simulink library "MX_Library"  (Simulink 7.7)
settings: Solver=ode45  StartTime=0.0  StopTime=10.0  RelTol=1e-3
values from neighbouring files (symbols this model uses):
  ACTIVE = Bobcat.Parameter; CreateDefine( ACTIVE                         ,1                          ,'Define' ,'defines.h' )    [defines.m]
  CD_PRECISION_REF_NOMINAL_VALUE = Bobcat.Parameter; CreateAliasCD( CD_PRECISION_REF_NOMINAL_VALUE                       ,uint16(511)                ,'ConstantDataPointer' ,'CONSTANT_DATA' ,'PRECISION_REF_NOMINAL_VALUE')    [cdata.m]
  ENGINE_CRANKING = Bobcat.Parameter; CreateDefine( ENGINE_CRANKING                ,2                          ,'Define' ,'defines.h' )    [defines.m]
  ERROR_OFF = Bobcat.Parameter; CreateDefine( ERROR_OFF                      ,3                          ,'Define' ,'defines.h' )    [defines.m]
  ERROR_ON = Bobcat.Parameter; CreateDefine( ERROR_ON                       ,2                          ,'Define' ,'defines.h' )    [defines.m]
  FAILURE = Bobcat.Parameter; CreateDefine( FAILURE                        ,28                         ,'Define' ,'defines.h' )    [defines.m]
  FULL_ON = Bobcat.Parameter; CreateDefine( FULL_ON                        ,fi(0,0,16,16,'hex','ffff') ,'Define' ,'defines.h' )    [defines.m]
  INACTIVE = Bobcat.Parameter; CreateDefine( INACTIVE                       ,0                          ,'Define' ,'defines.h' )    [defines.m]
  NON_FUNCTIONAL = Bobcat.Parameter; CreateDefine( NON_FUNCTIONAL                 ,255                        ,'Define' ,'defines.h' )    [defines.m]
  NORMAL = Bobcat.Parameter; CreateDefine( NORMAL                         ,8                          ,'Define' ,'defines.h' )    [defines.m]
  OORL = Bobcat.Parameter; CreateDefine( OORL                           ,22                         ,'Define' ,'defines.h' )    [defines.m]
  OPEN_CIRCUIT = Bobcat.Parameter; CreateDefine( OPEN_CIRCUIT                   ,7                          ,'Define' ,'defines.h' )    [defines.m]
  OPEN_STG = Bobcat.Parameter; CreateDefine( OPEN_STG                       ,31                         ,'Define' ,'defines.h' )    [defines.m]
  OVERCURRENT = Bobcat.Parameter; CreateDefine( OVERCURRENT                    ,32                         ,'Define' ,'defines.h' )    [defines.m]
  RESET = Bobcat.Parameter; CreateDefine( RESET                          ,2                          ,'Define' ,'defines.h' )    [defines.m]
  SHORT_TO_BATTERY = Bobcat.Parameter; CreateDefine( SHORT_TO_BATTERY               ,5                          ,'Define' ,'defines.h' )    [defines.m]
  SHORT_TO_GROUND = Bobcat.Parameter; CreateDefine( SHORT_TO_GROUND                ,6                          ,'Define' ,'defines.h' )    [defines.m]
  srate = 0.010    (= 0.01)    [LoadWorkspace.m]
  UNLIMITED = Bobcat.Parameter; CreateDefine( UNLIMITED                      ,65535                      ,'Define' ,'defines.h' )    [defines.m]
undefined symbols (not defined in the file or in its folder): BIDIRECTIONAL_CTRL, CD__AFBK_GAIN, CD__DEBOUNCE_OPEN_CIRCUIT, CD__DEBOUNCE_OVERCURRENT, CD__DEBOUNCE_SHORT_TO_BATTERY, CD__DEBOUNCE_SHORT_TO_GROUND, CD__ENABLE_AFBK_GAIN, CD__ENABLE_DEBOUNCE_OPEN_CIRCUIT, CD__ENABLE_DEBOUNCE_OVERCURRENT, CD__ENABLE_DEBOUNCE_SHORT_TO_BATTERY, CD__ENABLE_DEBOUNCE_SHORT_TO_GROUND, CD__ENABLE_FEEDBACK_FUNCTION, CD__ENABLE_IFBK_GAIN, CD__ENABLE_MAX_VOLTS, CD__ENABLE_NON_ZERO_CURRENT, CD__ENABLE_NON_ZERO_DUTY, CD__ENABLE_OVERCURRENT, CD__FUNCTION, CD__IFBK_GAIN, CD__KI, CD__KP, CD__MAX_VOLTS, CD__NON_ZERO_CURRENT, CD__NON_ZERO_DUTY, CD__OVERCURRENT, DEBOUNCE_ERROR_OFF, DEBOUNCE_ERROR_ON, DiscIntNeverNeededParam, FN_, IFBK_MAX, KI, KP, MAX_VOLTS, NZ_DUTY, NZ_IFBK, OC_DB_CNT, OPEN_DB_CNT, OSTG_DB_CNT, STB_DB_CNT, STG_DB_CNT
libraries: simulink x12, MX_Library x11
(part 2 of 2)

== stateflow chart oc_stg_detection/oc_operation_detection ==
  state NORMAL
    en:diag_state_out = NORMAL;
    en:ocstg_check = INACTIVE;
  state OC_STATE_ERROR
    en:diag_state_out = oc_state;
    en:ocstg_check = INACTIVE;
  state OPEN_STG_ERROR_RESET
    en:diag_state_out = NORMAL;
    en:ocstg_check = ACTIVE;
  state OPEN_STG_ERROR
    du:diag_state_out = diag_state_in;
    en:ocstg_check = INACTIVE;
    en:debounceCount = 0;
    (junction 157) -> (junction 158) : [(diag_state_in == NORMAL)]{debounceCount++;}
    OPEN_STG_ERROR -> (junction 157) [order 1]
  state DIAG_STATE_ERROR
    en:diag_state_out = diag_state_in;
    en:ocstg_check = INACTIVE;
  state OPEN_STG_DIAG_STATE
    en:ocstg_check = INACTIVE;
  state OPEN_STG_RESET
    en:ocstg_check = RESET;
  note: Pulse ocstg_check to reset fault state
      | to normal with output forced off to determine
      | if the fault is STG or Open Circuit
  note: During this state, lo-side is to enabled for a period of time to determine
      | if fault is open circuit.  Then lo-side is to be turned off to check for
      | short to ground.
  note: Error no longer detectable,
      | send reset to turn the output back on.
  (default) -> NORMAL
  NORMAL -> OPEN_STG_ERROR_RESET [order 1] : %Unable to distinguish
      | % between Open or STG fault
      | [(diag_state_in == OPEN_STG)]
  NORMAL -> OC_STATE_ERROR [order 2] : %Overcurrent Fault
      | [(oc_state != NORMAL)]
  OPEN_STG_DIAG_STATE -> OPEN_STG_ERROR : [after(5,tick)]
  NORMAL -> DIAG_STATE_ERROR [order 3] : %STB, STG or Open Circuit Fault
      | [(diag_state_in == SHORT_TO_GROUND)...
      | || (diag_state_in == SHORT_TO_BATTERY)...
      | || (diag_state_in == OPEN_CIRCUIT)]
  OPEN_STG_ERROR_RESET -> OPEN_STG_DIAG_STATE : [after(5,tick)]
  OPEN_STG_RESET -> NORMAL : [after(50,tick)]
  OPEN_STG_ERROR -> OPEN_STG_RESET [order 1] : [(debounceCount >= (OPEN_DB_CNT...
      | + STG_DB_CNT + 100))]
  data: oc_state input uint8; diag_state_in input uint8; diag_state_out output uint8; ocstg_check output uint8; ACTIVE parameter uint8; INACTIVE parameter uint8; OPEN_CIRCUIT parameter uint8; SHORT_TO_GROUND parameter uint8; SHORT_TO_BATTERY parameter uint8; OPEN_STG parameter uint8; NORMAL parameter uint8; debounceCount local uint16; RESET parameter uint8; OPEN_DB_CNT parameter uint16; STG_DB_CNT parameter uint16

== stateflow chart output_pair_ClosedLoop/control ==
  state DIAG_CHECK
    en:icmd_Out = INACTIVE;
    state ENABLE_ON
      en:enable_LoSide = ACTIVE;
      en:debounceCount = 0;
      du:debounceCount++;
    state ENABLE_OFF
      en:enable_LoSide = INACTIVE;
    note: Turns on the low side
        | (may take up to 0.5 sec for low side to actually
        | turn on due to delay in output enable function).
        | So, it is possible to detect STG right away
        | while in this state.
    note: Forces the low side off for STG detection
        | assuming it didn't detect it already while
        | waiting for the low side to turn on.
    note: To detect open circuit, low side must be on.
        | To detect STG, low side must be off.
    (default) -> ENABLE_ON
    ENABLE_ON -> ENABLE_OFF : %Give it some time to ensure low side is on
        | %and detect open circuit
        | [(debounceCount >= OPEN_DB_CNT + 100)]
  state ERROR
    en:
    icmd_Out = INACTIVE;
    enable_LoSide = INACTIVE;
    state_Output = diag_state;
  state FUNCTIONAL
    state STGOFF_DIAG_ACTIVE
      en:icmd_Out = INACTIVE;
      en:state_Output = INACTIVE;
      state Test_OC
        en:debounceCount = 0;
        en:enable_LoSide = ACTIVE;
        du:debounceCount++;
      state Test_STG
        en:debounceCount = 0;
        en:enable_LoSide = INACTIVE;
        du:debounceCount++;
      note: Testing for open circuit will turn on the low side
          | (may take up to 0.5 sec for low side to actually
          | turn on due to delay in output enable function).
          | So, it is possible to detect STG right away
          | while in this state.
      note: Forces the low side off for STG detection
          | assuming it didn't detect it already while
          | waiting for the low side to turn on.
      (default) -> Test_OC
      Test_STG -> Test_OC : [(debounceCount >= STG_DB_CNT + 100)]
      Test_OC -> Test_STG : [(debounceCount >= OPEN_DB_CNT + 100)]
    state STGOFF_DIAG_INACTIVE
      en:enable_LoSide = ACTIVE;
      state ACTIVE_ON
        en:icmd_Out = icmd_In;
        du:icmd_Out = icmd_In;
        en:state_Output = ACTIVE;
      state ACTIVE_OFF
        en:icmd_Out = INACTIVE;
        en:state_Output = INACTIVE;
      (default) -> ACTIVE_OFF
      ACTIVE_ON -> ACTIVE_OFF : [icmd_In == 0]
      ACTIVE_OFF -> ACTIVE_ON : [icmd_In > 0]
    note: Short to Ground detection is available
        | while hi side output is off by turning
        | off low-side periodically.
    note: Short to Ground detection is
        | not available while hi side output
        | is off
    STGOFF_DIAG_ACTIVE -> STGOFF_DIAG_INACTIVE : [!enable_STGOffDiag]
    STGOFF_DIAG_INACTIVE -> STGOFF_DIAG_ACTIVE : [enable_STGOffDiag]
    (default) -> STGOFF_DIAG_ACTIVE
  DIAG_CHECK -> FUNCTIONAL [order 1] : %Couldn't find a fault, so go back to working
      | %?? should this condition really be recoverable??
      | [(ocstg_check == RESET)]
  FUNCTIONAL -> DIAG_CHECK [order 2] : %Open or STG Fault detected
      | %while output is on
      | [(ocstg_check == ACTIVE)]
  (default) -> FUNCTIONAL
  DIAG_CHECK -> ERROR [order 2] : %Fault Detected
      | [(diag_state != NORMAL)]
  FUNCTIONAL -> ERROR [order 1] : %Fault Detected
      | [(diag_state != NORMAL)]
  data: state_Output output uint8; icmd_In input fixdt(0,16,12); icmd_Out output fixdt(0,16,12); enable_LoSide output boolean; ocstg_check input uint8; debounceCount local uint16 =0; ACTIVE parameter uint8; INACTIVE parameter uint8; RESET parameter uint8; diag_state input uint8; NORMAL parameter uint8; OPEN_DB_CNT parameter uint16; STG_DB_CNT parameter uint16; enable_STGOffDiag input boolean

== stateflow chart output_single_OpenLoop/control ==
  state ERROR
    en:duty_Output = INACTIVE;
    en:state_Output = error_Output;
  state FUNCTIONAL
    en:
    duty_Output = cmd_Output;
    du:
    duty_Output = cmd_Output;
    state ACTIVE
      en:
      state_Output = ACTIVE;
    state INACTIVE
      en:
      state_Output = INACTIVE;
    INACTIVE -> ACTIVE : [cmd_Output != INACTIVE]
    (default) -> INACTIVE
    ACTIVE -> INACTIVE : [cmd_Output == INACTIVE]
  FUNCTIONAL -> ERROR : [(error_Output != NORMAL)]
  ERROR -> FUNCTIONAL : [(error_Output == NORMAL)]
  (default) -> FUNCTIONAL
  data: duty_Output output fixdt(0,16,16); state_Output output uint8; cmd_Output input fixdt(0,16,16); error_Output input uint8; INACTIVE parameter uint8 =0; ACTIVE parameter uint8 =1; NORMAL parameter uint8

== stateflow chart output_pair_OpenLoop/control ==
  state DIAG_CHECK
    en:duty_Output = INACTIVE;
    state ENABLE_ON
      en:enable_LoSide = ACTIVE;
      en:debounceCount = 0;
      du:debounceCount++;
    state ENABLE_OFF
      en:enable_LoSide = INACTIVE;
    note: Turns on the low side
        | (may take up to 0.5 sec for low side to actually
        | turn on due to delay in output enable function).
        | So, it is possible to detect STG right away
        | while in this state.
    note: Forces the low side off for STG detection
        | assuming it didn't detect it already while
        | waiting for the low side to turn on.
    note: To detect open circuit, low side must be on.
        | To detect STG, low side must be off.
    (default) -> ENABLE_ON
    ENABLE_ON -> ENABLE_OFF : %Give it some time to ensure low side is on
        | %and detect open circuit
        | [(debounceCount >= OPEN_DB_CNT + 100)]
  state ERROR
    en:
    duty_Output = INACTIVE;
    enable_LoSide = INACTIVE;
    state_Output = diag_state;
  state FUNCTIONAL
    state STGOFF_DIAG_ACTIVE
      en:duty_Output = INACTIVE;
      en:state_Output = INACTIVE;
      state Test_OC
        en:debounceCount = 0;
        en:enable_LoSide = ACTIVE;
        du:debounceCount++;
      state Test_STG
        en:debounceCount = 0;
        en:enable_LoSide = INACTIVE;
        du:debounceCount++;
      note: Testing for open circuit will turn on the low side
          | (may take up to 0.5 sec for low side to actually
          | turn on due to delay in output enable function).
          | So, it is possible to detect STG right away
          | while in this state.
      note: Forces the low side off for STG detection
          | assuming it didn't detect it already while
          | waiting for the low side to turn on.
      (default) -> Test_OC
      Test_STG -> Test_OC : [(debounceCount >= STG_DB_CNT + 100)]
      Test_OC -> Test_STG : [(debounceCount >= OPEN_DB_CNT + 100)]
    state STGOFF_DIAG_INACTIVE
      en:enable_LoSide = ACTIVE;
      state ACTIVE_ON
        en:duty_Output = FULL_ON;
        en:state_Output = ACTIVE;
      state ACTIVE_OFF
        en:duty_Output = INACTIVE;
        en:state_Output = INACTIVE;
      (default) -> ACTIVE_OFF
      ACTIVE_ON -> ACTIVE_OFF : [(cmd_Output != ACTIVE)]
      ACTIVE_OFF -> ACTIVE_ON : [(cmd_Output == ACTIVE)]
    note: Short to Ground detection is available
        | while hi side output is off by turning
        | off low-side periodically.
    note: Short to Ground detection is
        | not available while hi side output
        | is off
    STGOFF_DIAG_ACTIVE -> STGOFF_DIAG_INACTIVE : [!enable_STGOffDiag]
    STGOFF_DIAG_INACTIVE -> STGOFF_DIAG_ACTIVE : [enable_STGOffDiag]
    (default) -> STGOFF_DIAG_ACTIVE
  DIAG_CHECK -> FUNCTIONAL [order 1] : %Couldn't find a fault, so go back to working
      | %?? should this condition really be recoverable??
      | [(ocstg_check == RESET)]
  FUNCTIONAL -> DIAG_CHECK [order 2] : %Open or STG Fault detected
      | %while output is on
      | [(ocstg_check == ACTIVE)]
  (default) -> FUNCTIONAL
  DIAG_CHECK -> ERROR [order 2] : %Fault Detected
      | [(diag_state != NORMAL)]
  FUNCTIONAL -> ERROR [order 1] : %Fault Detected
      | [(diag_state != NORMAL)]
  ERROR -> FUNCTIONAL : [(diag_state == NORMAL)]
  data: state_Output output uint8; cmd_Output input boolean; enable_STGOffDiag input boolean; duty_Output output fixdt(0,16,16); enable_LoSide output boolean; ocstg_check input uint8; debounceCount local uint16 =0; ACTIVE parameter uint8; INACTIVE parameter uint8; RESET parameter uint8; diag_state input uint8; NORMAL parameter uint8; OPEN_DB_CNT parameter uint16; STG_DB_CNT parameter uint16; FULL_ON parameter fixdt(0,16,16)

== stateflow chart dout_chk/Fault monitor ==
  state diagnostics
    during: os=out_state();
    state Ok
      en: state = 8;
    state error
      en: state=os;
    state debounce
    state y=out_state [function]
      (default) -> (junction 314)
      (junction 314) -> (junction 315) : {
          | /* command, off feedback, on */
          | aVarTruthTableCondition_1 = (cmd==0 && fbk==1);
          | }
      (junction 315) -> (junction 316) : {
          | /* command, on feedback, off */
          | aVarTruthTableCondition_2 = (cmd==1 && fbk==0);
          | }
      (junction 316) -> (junction 317) [order 1] : [aVarTruthTableCondition_1]
      (junction 317) -> (junction 318) : {
          | /* 'E_on':Error On */
          | y=2; db_limit=ERR_ON_DB_CNT;
          | }
      (junction 316) -> (junction 319) [order 2]
      (junction 319) -> (junction 320) [order 1] : [aVarTruthTableCondition_2]
      (junction 320) -> (junction 321) : {
          | /* 'E_off':Error Off */
          | y=3; db_limit=ERR_OFF_DB_CNT;
          | }
      (junction 319) -> (junction 322) [order 2]
      (junction 322) -> (junction 323) : /* Default */
      (junction 323) -> (junction 324) : {
          | /* 'ok':default */
          | y=8;
          | }
    (default) -> Ok
    debounce -> error [order 2] : [db_cnt >= db_limit]
    debounce -> (junction 313) [order 3]
    debounce -> Ok [order 1] : [db_cnt==0]
    Ok -> debounce : [os!=8]/
        | db_state=os;
        | db_cnt++;
    (junction 312) -> debounce [order 2] : {db_cnt=1;
        | db_state=os}
    (junction 313) -> debounce [order 1] : [db_state==os]/
        | db_cnt++;
    (junction 313) -> (junction 312) [order 2]
    (junction 312) -> debounce [order 1] : [os==8]/
        | db_cnt--;
  data: os local uint8; db_cnt local uint16; db_state local uint8; db_limit local uint16 =20; y function_output uint8; aVarTruthTableCondition_1 temporary boolean =0; aVarTruthTableCondition_2 temporary boolean =0; cmd input boolean; fbk input boolean; state output uint8; ERR_ON_DB_CNT parameter uint16; ERR_OFF_DB_CNT parameter uint16
  data aVarTruthTableCondition_1 settings: description=|
      | command, off
      | feedback, on
  data aVarTruthTableCondition_2 settings: description=|
      | command, on
      | feedback, off

== stateflow chart Remove_OOR_Levels/RemoveOORLevels ==
  (default) -> (junction 359)
  (junction 359) -> (junction 360) [order 1] : [(fltValue_in > OORL_LEVEL)...
      | && (fltValue_in < OORH_LEVEL)]
  (junction 360) -> (junction 361) : {
      | fltValue_out = fltValue_in;
      | fltValue_old = fltValue_in;
      | }
  (junction 361) -> (junction 362)
  (junction 359) -> (junction 362) [order 2] : {
      | fltValue_out = fltValue_old;
      | }
  data: fltValue_in input uint16; fltValue_out output uint16; fltValue_old local uint16 =0; OORL_LEVEL parameter uint16; OORH_LEVEL parameter uint16

== stateflow chart hc_pair_OpenLoop/Open_Loop/Fault monitor ==
  state FAULT [parallel]
    settings: executionOrder=2
    state ACTIVE
      state OC_STG
        state FAULT
          en:diag_state = OPEN_STG;
        state DEBOUNCE
          en: db_cnt = 0;
          du: db_cnt++;
        FAULT.ACTIVE.OC_STG.DEBOUNCE -> FAULT.ACTIVE.OC_STG.FAULT : [(db_cnt >= OSTG_DB_CNT)]
        (default) -> FAULT.ACTIVE.OC_STG.DEBOUNCE
      state NORMAL
        en: diag_state = NORMAL;
        en: db_cnt = 0;
      state OPEN_CIRCUIT
        state DEBOUNCE
          en: db_cnt = 0;
          du: db_cnt++;
        state FAULT
          en:diag_state = OPEN_CIRCUIT;
        FAULT.ACTIVE.OPEN_CIRCUIT.DEBOUNCE -> FAULT.ACTIVE.OPEN_CIRCUIT.FAULT : [(db_cnt >= OPEN_DB_CNT)]
        (default) -> FAULT.ACTIVE.OPEN_CIRCUIT.DEBOUNCE
      state SHORT_TO_GROUND
        state DEBOUNCE
          en: db_cnt = 0;
          du: db_cnt++;
        state FAULT
          en:diag_state = SHORT_TO_GROUND;
        FAULT.ACTIVE.SHORT_TO_GROUND.DEBOUNCE -> FAULT.ACTIVE.SHORT_TO_GROUND.FAULT : [(db_cnt >= STG_DB_CNT)]
        (default) -> FAULT.ACTIVE.SHORT_TO_GROUND.DEBOUNCE
      state SHORT_TO_BATTERY
        state FAULT
          en:diag_state = SHORT_TO_BATTERY;
        state DEBOUNCE
          en: db_cnt = 0;
          du: db_cnt++;
        FAULT.ACTIVE.SHORT_TO_BATTERY.DEBOUNCE -> FAULT.ACTIVE.SHORT_TO_BATTERY.FAULT : [(db_cnt >= STB_DB_CNT)]
        (default) -> FAULT.ACTIVE.SHORT_TO_BATTERY.DEBOUNCE
      note: With high side on, can't distinguish between
          | an open circuit or short to ground
      (default) -> FAULT.ACTIVE.NORMAL
      FAULT.ACTIVE.NORMAL -> SHORT_TO_BATTERY [order 1] : [(hs_cmd == INACTIVE)...
          | && (afbk_ratio > 0.80C)...
          | && (diag_enable)]
      OC_STG -> FAULT.ACTIVE.NORMAL : [(diag_state == NORMAL)...
          | && (!(ls_cmd)...
          |         || (hs_cmd <= NZ_DUTY)...
          |         || (ifbk > NZ_IFBK)...
          |         || !(diag_enable))]
      SHORT_TO_GROUND -> FAULT.ACTIVE.NORMAL : [(diag_state == NORMAL)...
          | && ((ls_cmd)...
          |         || (afbk_ratio >= 0.20C)...
          |         || !(diag_enable))]
      FAULT.ACTIVE.NORMAL -> SHORT_TO_GROUND [order 4] : [!(ls_cmd)...
          | && (afbk_ratio < 0.20C)...
          | && (diag_enable)]
      OPEN_CIRCUIT -> FAULT.ACTIVE.NORMAL : [(diag_state == NORMAL)...
          | && ((hs_cmd != INACTIVE)...
          |        || !(ls_cmd)...
          |        || (afbk_ratio <= 0.25C)...
          |        || (afbk_ratio >= 0.75C)...
          |        || !(diag_enable))]
      FAULT.ACTIVE.NORMAL -> OPEN_CIRCUIT [order 3] : [(hs_cmd == INACTIVE)...
          | && (ls_cmd)...
          | && (afbk_ratio > 0.25C)...
          | && (afbk_ratio < 0.75C)...
          | && (diag_enable)]
      FAULT.ACTIVE.NORMAL -> OC_STG [order 2] : [(ls_cmd)...
          | && (hs_cmd > NZ_DUTY)...
          | && (ifbk <= NZ_IFBK)...
          | && (diag_enable)]
      SHORT_TO_BATTERY -> FAULT.ACTIVE.NORMAL : [(diag_state == NORMAL)...
          | && ((hs_cmd != INACTIVE)...
          |         || (afbk_ratio <= 0.80C)...
          |         || !(diag_enable))]
    state INACTIVE
      en: diag_state = NORMAL;
    (default) -> INACTIVE
    INACTIVE -> ACTIVE : [ocstg_check != ACTIVE]
    ACTIVE -> INACTIVE : [ocstg_check == ACTIVE]
  state OUTPUT [parallel]
    settings: executionOrder=1
    state OFF
      en: hs_cmd = INACTIVE;
      en: ls_cmd = INACTIVE;
    state TURNING_OFF
      en: hs_cmd = INACTIVE;
    state TURNING_ON
      en: ls_cmd = ACTIVE;
    state ON
      du: hs_cmd = duty;
    (default) -> OFF
    ON -> OFF [order 2] : [(oc_state == OVERCURRENT)]
    TURNING_OFF -> OFF : [after(2, tick)]
    (junction 401) -> TURNING_ON : [(enable == ACTIVE)...
        | && (oc_state == NORMAL)...
        | && (diag_enable == ACTIVE)]
    ON -> TURNING_OFF [order 1] : [(enable == INACTIVE)...
        | || (diag_enable == INACTIVE)]
    TURNING_ON -> ON : [after(2, tick)]
    OFF -> (junction 401) : [after(50, tick)]
  state OVERCURRENT [parallel]
    settings: executionOrder=3
    state NORMAL
      en:oc_state = NORMAL;
      en:db_cnt_oc = 0;
    state debounce
      du: db_cnt_oc++;
    state error
      entry: oc_state = OVERCURRENT;
      du: hs_cmd = INACTIVE;
      du: ls_cmd = INACTIVE;
    debounce -> error [order 1] : [(db_cnt_oc >=OC_DB_CNT)]
    (default) -> OVERCURRENT.NORMAL
    OVERCURRENT.NORMAL -> debounce : [(ifbk > IFBK_MAX)...
        | && (diag_enable)]
        | {
        | db_cnt_oc++;
        | }
    debounce -> OVERCURRENT.NORMAL [order 2] : [(ifbk <= IFBK_MAX)...
        | || !(diag_enable)]
  data: duty input double; hs_cmd output fixdt(0,16,16); ls_cmd output boolean; diag_state output uint8 =8; afbk_ratio input fixdt(1,16,8); ifbk input fixdt(0,16,12); NZ_IFBK parameter fixdt(0,16,12); NZ_DUTY parameter fixdt(0,16,16); ocstg_check input uint8; STB_DB_CNT parameter uint16; OPEN_DB_CNT parameter uint16; OSTG_DB_CNT parameter uint16; STG_DB_CNT parameter uint16; db_cnt local uint16; enable input boolean; oc_state output uint8; IFBK_MAX parameter fixdt(0,16,12); OC_DB_CNT parameter uint16; db_cnt_oc local uint16; ACTIVE parameter uint8; INACTIVE parameter uint8; NORMAL parameter uint8; OVERCURRENT parameter uint8; SHORT_TO_GROUND parameter uint8; SHORT_TO_BATTERY parameter uint8; OPEN_CIRCUIT parameter uint8; OPEN_STG parameter uint8; diag_enable input boolean
